simulink model "Senorless"  (R2023a)
settings: Solver=FixedStepDiscrete  StartTime=0.0  StopTime=2  FixedStep=1/FOC_FRQ  RelTol=1e-3
values from neighbouring files (symbols this model uses):
  ADC_REF = 3.6    [Senorless.sldd]
  ADC_SAMPLE_MAX = 32767.0    [Senorless.sldd]
  AMP_GAIN = 32.0    [Senorless.sldd]
  CURR_INPUT = 3276.0    [Senorless.sldd]
  CURR_KI = 380.0    [Senorless.sldd]
  CURR_KP = 0.04    [Senorless.sldd]
  CURR_LIMIT = 1.1    [Senorless.sldd]
  CURR_OVER = 34.0    [Senorless.sldd]
  CURR_POINT_GAIN = 7.0    [Senorless.sldd]
  CURR_STEP = 32760.0    [Senorless.sldd]
  CURR_UNDER = 0.03    [Senorless.sldd]
  CURR_WIDTH = 250.0    [Senorless.sldd]
  FOC_FRQ = 36000.0    [Senorless.sldd]
  GAMMA = 32767.0    [Senorless.sldd]
  HFI_ID = 2.125    [Senorless.sldd]
  IMAX = 34.0    [Senorless.sldd]
  LPF_FRQ = 300.0    [Senorless.sldd]
  MOTOR_DAMPER = 8.3E-7    [Senorless.sldd]
  MOTOR_FLUX = 0.0012713112    [Senorless.sldd]
  MOTOR_INERTIA = 1.02E-6    [Senorless.sldd]
  MOTOR_LS = 1.8E-5    [Senorless.sldd]
  MOTOR_PN = 7.0    [Senorless.sldd]
  MOTOR_RS = 0.065    [Senorless.sldd]
  NS_COMP_UD = 0.531    [Senorless.sldd]
  PLL_LIMIT = 0.95    [Senorless.sldd]
  PLL_WIDTH = 500.0    [Senorless.sldd]
  PWM_FRQ = 96000000.0    [Senorless.sldd]
  RS_HUNT = 0.002    [Senorless.sldd]
  SMOK_FRQ = 1200.0    [Senorless.sldd]
  SPD_LIMIT = 0.8    [Senorless.sldd]
  SPD_LPF_LEVEL = 15.0    [Senorless.sldd]
  SPD_MAX = 8100.0    [Senorless.sldd]
  SPD_MIN = -8100.0    [Senorless.sldd]
  SPD_REDUCE = 380.0    [Senorless.sldd]
  SPD_STEP = 3.0    [Senorless.sldd]
  SPD_WIDTH = 10.0    [Senorless.sldd]
  TS_POINT_GAIN = 10.0    [Senorless.sldd]
  UDC = 17.0    [Senorless.sldd]
  UDC_GAIN = 21.0    [Senorless.sldd]
  UDC_POINT_GAIN = 10.0    [Senorless.sldd]
undefined symbols (not defined in the file or in its folder): curr_q_ki, curr_q_kp, DiscIntNeverNeededParam, magnitude, PLL_LPF_LEVEL, Udc
libraries: simulink x20, slpidlib x5, mcbcontrolslib x4, mcbplantlib x1, autolibpmsminterior x1, autolibpmsmexterior x1, spspowerguiLib x1
(part 2 of 7)

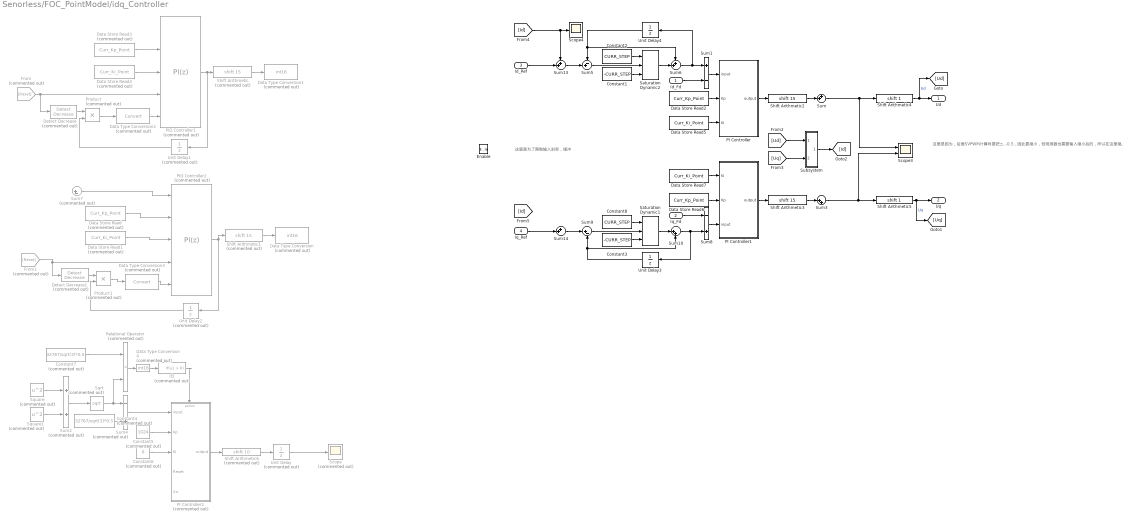
== system Senorless/FOC_PointModel/idq_Controller ==
  note: 这里是为了限制输入斜率，缓冲
  note: 这里是因为，后面SVPWM计算时要把±1映射去±0.5，因此要缩小，但观测器也需要输入缩小后的，所以在这里缩。
  Id_Fd : Inport
  Iq_Fd : Inport  Port=2
  Id_Ref : Inport  Port=3
  Iq_Ref : Inport  Port=4
  Enable : EnablePort  StatesWhenEnabling=reset  PropagateVarSize=During execution
  Constant1 : Constant  Value=-CURR_STEP  OutDataTypeStr=int16
  Constant2 : Constant  Value=CURR_STEP  OutDataTypeStr=int16
  Constant3 : Constant  Value=-CURR_STEP  OutDataTypeStr=int16
  Constant4 : Constant  Commented=on  Value=32767/sqrt(3)*0.5  OutDataTypeStr=int32
  Constant5 : Constant  Commented=on  Value=1024  OutDataTypeStr=int16
  Constant6 : Constant  Commented=on  Value=0  OutDataTypeStr=int16
  Constant7 : Constant  Commented=on  Value=32767/sqrt(3)*0.5  OutDataTypeStr=int32
  Constant8 : Constant  Value=CURR_STEP  OutDataTypeStr=int16
  Data Store Read : DataStoreRead  Commented=on  DataStoreName=Curr_Kp_Point  IndexOptions=Index vector (dialog)  Indices=1  OutputSizes=1
  Data Store Read1 : DataStoreRead  Commented=on  DataStoreName=Curr_Ki_Point  IndexOptions=Index vector (dialog)  Indices=1  OutputSizes=1
  Data Store Read2 : DataStoreRead  DataStoreName=Curr_Kp_Point  IndexOptions=Index vector (dialog)  Indices=1  OutputSizes=1
  Data Store Read3 : DataStoreRead  Commented=on  DataStoreName=Curr_Kp_Point  IndexOptions=Index vector (dialog)  Indices=1  OutputSizes=1
  Data Store Read4 : DataStoreRead  Commented=on  DataStoreName=Curr_Ki_Point  IndexOptions=Index vector (dialog)  Indices=1  OutputSizes=1
  Data Store Read5 : DataStoreRead  DataStoreName=Curr_Ki_Point  IndexOptions=Index vector (dialog)  Indices=1  OutputSizes=1
  Data Store Read6 : DataStoreRead  DataStoreName=Curr_Kp_Point  IndexOptions=Index vector (dialog)  Indices=1  OutputSizes=1
  Data Store Read7 : DataStoreRead  DataStoreName=Curr_Ki_Point  IndexOptions=Index vector (dialog)  Indices=1  OutputSizes=1
  Data Type Conversion : DataTypeConversion  Commented=on  OutDataTypeStr=int16  SaturateOnIntegerOverflow=off  RndMeth=Floor
  Data Type Conversion1 : DataTypeConversion  Commented=on  OutDataTypeStr=int16  SaturateOnIntegerOverflow=off  RndMeth=Floor
  Data Type Conversion2 : DataTypeConversion  Commented=on  SaturateOnIntegerOverflow=off  RndMeth=Floor
  Data Type Conversion3 : DataTypeConversion  Commented=on  SaturateOnIntegerOverflow=off  RndMeth=Floor
  Data Type Conversion4 : DataTypeConversion  Commented=on  OutDataTypeStr=int16  SaturateOnIntegerOverflow=off
  Detect Decrease : simulink/Logic and Bit Operations/Detect Decrease  Commented=on  vinit=0.0  OutDataTypeStr=uint8
  Detect Decrease1 : simulink/Logic and Bit Operations/Detect Decrease  Commented=on  vinit=0.0  OutDataTypeStr=uint8
  From : From  Commented=on  GotoTag=Reset
  From1 : From  Commented=on  GotoTag=Reset
  If2 : If  Commented=on  ShowElse=off
  PI Controller : Subsystem
      settings: MinAlgLoopOccurrences=on
  PI Controller1 : Subsystem
      settings: MinAlgLoopOccurrences=on
  PI Controller2 : Subsystem  Commented=on  TreatAsAtomicUnit=on
      settings: MinAlgLoopOccurrences=on
  PID Controller1 : slpidlib/PID Controller  Commented=on  Controller=PI  Form=Parallel  TimeDomain=Discrete-time  UseExternalTs=off  SampleTime=-1  IntegratorMethod=Forward Euler  FilterMethod=Forward Euler  ControllerParametersSource=external  P=curr_q_kp  I=curr_q_ki  UseKiTs=off  D=0  N=100  UseFilter=on  TunerSelectOption=Transfer Function Based (PID Tuner App)  ZeroCross=off  InitialConditionSource=external  InitialConditionForIntegrator=0  InitialConditionForFilter=0  DifferentiatorICPrevScaledInput=0  ExternalReset=either  TrackingMode=off  Kt=1  LimitOutput=on  SatLimitsSource=internal  UpperSaturationLimit=32767*32767  LowerSaturationLimit=-32767*32767  LinearizeAsGain=on  AntiWindupMode=clamping  Kb=1  LimitIntegrator=on  UpperIntegratorSaturationLimit=32767*32767  LowerIntegratorSaturationLimit=-32767*32767  RndMeth=Zero  SaturateOnIntegerOverflow=on  PGainOutDataTypeStr=int32  PProdOutDataTypeStr=int32  POutMin=[]  POutMax=[]  IGainOutDataTypeStr=int32  IProdOutDataTypeStr=int32  IOutMin=[]  IOutMax=[]  DOutMin=[]  DOutMax=[]  NOutMin=[]  NOutMax=[]  SumOutDataTypeStr=int32  SumOutMin=[]  SumOutMax=[]  SaturationOutDataTypeStr=int32  SaturationOutMin=[]  SaturationOutMax=[]  PParamMin=[]  PParamMax=[]  IParamMin=[]  IParamMax=[]  DParamMin=[]  DParamMax=[]  NParamMin=[]  NParamMax=[]  KbParamMin=[]  KbParamMax=[]  KtParamMin=[]  KtParamMax=[]  KbOutMin=[]  KbOutMax=[]  KtOutMin=[]  KtOutMax=[]  IntegratorOutDataTypeStr=int32  IntegratorOutMin=[]  IntegratorOutMax=[]  FilterOutMin=[]  FilterOutMax=[]  SumI1OutMin=[]  SumI1OutMax=[]  SumI2OutMin=[]  SumI2OutMax=[]  SumI3OutMin=[]  SumI3OutMax=[]  SumI4OutMin=[]  SumI4OutMax=[]  SumDOutMin=[]  SumDOutMax=[]  SumAccumDataTypeStr=int32  DifferentiatorOutMin=[]  DifferentiatorOutMax=[]  FilterDiffOutCoefMin=[]  FilterDiffOutCoefMax=[]  ReciprocalOutMin=[]  ReciprocalOutMax=[]  SumDenOutMin=[]  SumDenOutMax=[]  SumNumOutMin=[]  SumNumOutMax=[]  DivideOutMin=[]  DivideOutMax=[]  UdiffTsProdOutMin=[]  UdiffTsProdOutMax=[]  NTsProdOutMin=[]  NTsProdOutMax=[]  UintegralTsProdOutMin=[]  UintegralTsProdOutMax=[]  UngainTsProdOutMin=[]  UngainTsProdOutMax=[]  ClampingZeroOutDataTypeStr=int32  ClampingZeroOutMin=[]  ClampingZeroOutMax=[]  FilterDenConstantOutDataTypeStr=Inherit: Inherit via back propagation  FilterDenConstantOutMin=[]  FilterDenConstantOutMax=[]  PCopyOutDataTypeStr=Inherit: Inherit via back propagation  PCopyOutMin=[]  PCopyOutMax=[]  NCopyOutDataTypeStr=Inherit: Inherit via back propagation  NCopyOutMin=[]  NCopyOutMax=[]  IntegratorContinuousStateAttributes=''  IntegratorStateMustResolveToSignalObject=off  IntegratorRTWStateStorageClass=Auto  FilterContinuousStateAttributes=''  FilterStateMustResolveToSignalObject=off  FilterRTWStateStorageClass=Auto  ParallelPVariant=ExternalParameters  IdealPVariant=Disabled  IVariant=ExternalParameters  DVariant=Disabled  IntegratorVariant=Discrete  SatVariant=Enabled  AWVariant=DiscClampingParallel  PCopyVariant=Disabled  TRVariant=Disabled  FdbkBlocksVariant=Forward  IdealPFdbkVariant=Disabled  SatFdbkVariant=Disabled  DerivativeFilterVariant=Disabled  NVariant=Disabled  NCopyVariant=Disabled_SignalSpec  FilterICVariant=Disabled  IntegratorICVariant=ExternalICs  ExternalResetVariant=ExternalReset  TRSumVariant=Passthrough  SumFdbkVariant=Disabled  SumVariant=Sum_PI  TsampFilterVariant=InternalTs  TsampNgainVariant=Passthrough  TsampIntegralVariant=Disabled_SignalSpec  ExternalSaturationOutDataTypeStr=int32
  PID Controller2 : slpidlib/PID Controller  Commented=on  Controller=PI  Form=Parallel  TimeDomain=Discrete-time  UseExternalTs=off  SampleTime=-1  IntegratorMethod=Forward Euler  FilterMethod=Forward Euler  ControllerParametersSource=external  P=curr_q_kp  I=curr_q_ki  UseKiTs=off  D=0  N=100  UseFilter=on  TunerSelectOption=Transfer Function Based (PID Tuner App)  ZeroCross=off  InitialConditionSource=external  InitialConditionForIntegrator=0  InitialConditionForFilter=0  DifferentiatorICPrevScaledInput=0  ExternalReset=either  TrackingMode=off  Kt=1  LimitOutput=on  SatLimitsSource=internal  UpperSaturationLimit=32767*32767  LowerSaturationLimit=-32767*32767  LinearizeAsGain=on  AntiWindupMode=none  Kb=1  LimitIntegrator=on  UpperIntegratorSaturationLimit=32767*32767  LowerIntegratorSaturationLimit=-32767*32767  RndMeth=Zero  SaturateOnIntegerOverflow=on  PGainOutDataTypeStr=int32  PProdOutDataTypeStr=int32  POutMin=[]  POutMax=[]  IGainOutDataTypeStr=int32  IProdOutDataTypeStr=int32  IOutMin=[]  IOutMax=[]  DOutMin=[]  DOutMax=[]  NOutMin=[]  NOutMax=[]  SumOutDataTypeStr=int32  SumOutMin=[]  SumOutMax=[]  SaturationOutDataTypeStr=int32  SaturationOutMin=[]  SaturationOutMax=[]  PParamMin=[]  PParamMax=[]  IParamMin=[]  IParamMax=[]  DParamMin=[]  DParamMax=[]  NParamMin=[]  NParamMax=[]  KbParamMin=[]  KbParamMax=[]  KtParamMin=[]  KtParamMax=[]  KbOutMin=[]  KbOutMax=[]  KtOutMin=[]  KtOutMax=[]  IntegratorOutDataTypeStr=int32  IntegratorOutMin=[]  IntegratorOutMax=[]  FilterOutMin=[]  FilterOutMax=[]  SumI1OutMin=[]  SumI1OutMax=[]  SumI2OutMin=[]  SumI2OutMax=[]  SumI3OutMin=[]  SumI3OutMax=[]  SumI4OutMin=[]  SumI4OutMax=[]  SumDOutMin=[]  SumDOutMax=[]  SumAccumDataTypeStr=int32  DifferentiatorOutMin=[]  DifferentiatorOutMax=[]  FilterDiffOutCoefMin=[]  FilterDiffOutCoefMax=[]  ReciprocalOutMin=[]  ReciprocalOutMax=[]  SumDenOutMin=[]  SumDenOutMax=[]  SumNumOutMin=[]  SumNumOutMax=[]  DivideOutMin=[]  DivideOutMax=[]  UdiffTsProdOutMin=[]  UdiffTsProdOutMax=[]  NTsProdOutMin=[]  NTsProdOutMax=[]  UintegralTsProdOutMin=[]  UintegralTsProdOutMax=[]  UngainTsProdOutMin=[]  UngainTsProdOutMax=[]  ClampingZeroOutDataTypeStr=int32  ClampingZeroOutMin=[]  ClampingZeroOutMax=[]  FilterDenConstantOutDataTypeStr=Inherit: Inherit via back propagation  FilterDenConstantOutMin=[]  FilterDenConstantOutMax=[]  PCopyOutDataTypeStr=Inherit: Inherit via back propagation  PCopyOutMin=[]  PCopyOutMax=[]  NCopyOutDataTypeStr=Inherit: Inherit via back propagation  NCopyOutMin=[]  NCopyOutMax=[]  IntegratorContinuousStateAttributes=''  IntegratorStateMustResolveToSignalObject=off  IntegratorRTWStateStorageClass=Auto  FilterContinuousStateAttributes=''  FilterStateMustResolveToSignalObject=off  FilterRTWStateStorageClass=Auto  ParallelPVariant=ExternalParameters  IdealPVariant=Disabled  IVariant=ExternalParameters  DVariant=Disabled  IntegratorVariant=Discrete  SatVariant=Enabled  AWVariant=Passthrough  PCopyVariant=Disabled  TRVariant=Disabled  FdbkBlocksVariant=Forward  IdealPFdbkVariant=Disabled  SatFdbkVariant=Disabled  DerivativeFilterVariant=Disabled  NVariant=Disabled  NCopyVariant=Disabled_SignalSpec  FilterICVariant=Disabled  IntegratorICVariant=ExternalICs  ExternalResetVariant=ExternalReset  TRSumVariant=Passthrough  SumFdbkVariant=Disabled  SumVariant=Sum_PI  TsampFilterVariant=InternalTs  TsampNgainVariant=Passthrough  TsampIntegralVariant=Disabled_SignalSpec  ExternalSaturationOutDataTypeStr=int32
  Product : Product  Commented=on  OutDataTypeStr=int32  RndMeth=Zero
  Product1 : Product  Commented=on  OutDataTypeStr=int32  RndMeth=Zero
  Relational Operator : RelationalOperator  Commented=on  Operator=<  OutDataTypeStr=boolean  RndMeth=Zero  InputSameDT=off
  Saturation Dynamic1 : simulink/Discontinuities/Saturation Dynamic  OutMin=[]  OutMax=[]  OutDataTypeStr=Inherit: Same as second input  OutDataType=fixdt(1, 16)  OutScaling=2^-10  RndMeth=Zero  DoSatur=off
  Saturation Dynamic2 : simulink/Discontinuities/Saturation Dynamic  OutMin=[]  OutMax=[]  OutDataTypeStr=Inherit: Same as second input  OutDataType=fixdt(1, 16)  OutScaling=2^-10  RndMeth=Zero  DoSatur=off
  Scope : Scope  Commented=on
  Scope3 : Scope  NumInputPorts=2
  Scope4 : Scope
  Shift Arithmetic : ArithShift  Commented=on  BitShiftNumber=15
  Shift Arithmetic1 : ArithShift  Commented=on  BitShiftNumber=15
  Shift Arithmetic2 : ArithShift  BitShiftNumber=15
  Shift Arithmetic3 : ArithShift  BitShiftNumber=15
  Shift Arithmetic4 : ArithShift  BitShiftNumber=1
  Shift Arithmetic5 : ArithShift  BitShiftNumber=1
  Shift Arithmetic6 : ArithShift  Commented=on  BitShiftNumber=10
  Sqrt : Sqrt  Commented=on  OutputSignalType=real  RndMeth=Zero
  Square : Math  Commented=on  Operator=square
  Square1 : Math  Commented=on  Operator=square
  Subsystem : Subsystem
  Sum : Sum  Inputs=++|
  Sum1 : Sum  Inputs=+-  AccumDataTypeStr=int32  OutDataTypeStr=int32  RndMeth=Zero
  Sum10 : Sum  Inputs=|++  OutDataTypeStr=int16  RndMeth=Zero
  Sum13 : Sum  Inputs=++|  OutDataTypeStr=int16  RndMeth=Zero
  Sum14 : Sum  Inputs=++|  OutDataTypeStr=int16  RndMeth=Zero
  Sum2 : Sum  Commented=on  RndMeth=Zero
  Sum3 : Sum  Inputs=|++
  Sum4 : Sum  Commented=on  Inputs=-+  RndMeth=Zero
  Sum5 : Sum  Inputs=-+|  AccumDataTypeStr=int16  OutDataTypeStr=int16  RndMeth=Zero
  Sum6 : Sum  Inputs=++|  OutDataTypeStr=int16  RndMeth=Zero
  Sum7 : Sum  Commented=on  Inputs=|+-  AccumDataTypeStr=int32  OutDataTypeStr=int32  RndMeth=Zero
  Sum8 : Sum  Inputs=-+  AccumDataTypeStr=int32  OutDataTypeStr=int32  RndMeth=Zero
  Sum9 : Sum  Inputs=|+-  AccumDataTypeStr=int16  OutDataTypeStr=int16  RndMeth=Zero
  Unit Delay : UnitDelay  Commented=on  SampleTime=-1  HasFrameUpgradeWarning=on
  Unit Delay1 : UnitDelay  Commented=on  SampleTime=-1  HasFrameUpgradeWarning=on
  Unit Delay2 : UnitDelay  Commented=on  SampleTime=-1  HasFrameUpgradeWarning=on
  Unit Delay3 : UnitDelay  SampleTime=-1  HasFrameUpgradeWarning=on
  Unit Delay4 : UnitDelay  SampleTime=-1  HasFrameUpgradeWarning=on
  Ud : Outport  OutputWhenDisabled=reset  InitialOutput=int32(0)
  Uq : Outport  Port=2  OutputWhenDisabled=reset  InitialOutput=int32(0)
  wires:
  Sum7/1 -> PID Controller2/1
  Shift Arithmetic/1 -> Data Type Conversion1/1
  Shift Arithmetic1/1 -> Data Type Conversion/1
  Data Store Read/1 -> PID Controller2/2
  Data Store Read1/1 -> PID Controller2/3
  Data Store Read3/1 -> PID Controller1/2
  Data Store Read4/1 -> PID Controller1/3
  PID Controller1/1 -> Unit Delay1/1, Shift Arithmetic/1
  Unit Delay1/1 -> Product/2
  Detect Decrease/1 -> Product/1
  Product/1 -> Data Type Conversion2/1
  From/1 -> PID Controller1/4, Detect Decrease/1
  Unit Delay2/1 -> Product1/2
  Product1/1 -> Data Type Conversion3/1
  From1/1 -> PID Controller2/4, Detect Decrease1/1
  PID Controller2/1 -> Shift Arithmetic1/1, Unit Delay2/1
  Detect Decrease1/1 -> Product1/1
  Data Type Conversion3/1 -> PID Controller2/5
  PI Controller/1(output) -> Shift Arithmetic2/1
  Data Store Read5/1 -> PI Controller/3(Ki)
  Data Type Conversion2/1 -> PID Controller1/5
  Sum1/1 -> PI Controller/1(input)
  PI Controller1/1(output) -> Shift Arithmetic3/1
  Data Store Read2/1 -> PI Controller/2(Kp)
  Saturation Dynamic2/1 -> Sum6/2
  Unit Delay4/1 -> Sum6/1, Sum5/1
  Sum6/1 -> Unit Delay4/1, Sum1/1
  Constant1/1 -> Saturation Dynamic2/3
  Shift Arithmetic3/1 -> Sum3/1
  Shift Arithmetic4/1 -> [Ud], Ud/1  "Ud"
  Shift Arithmetic5/1 -> [Uq], Uq/1  "Uq"
  Square1/1 -> Sum2/2
  Square/1 -> Sum2/1
  Sum2/1 -> Sqrt/1
  Constant4/1 -> Sum4/2
  Sqrt/1 -> Relational Operator/2, Sum4/1
  Sum4/1 -> PI Controller2/1(input)
  Constant5/1 -> PI Controller2/2(Kp)
  Constant6/1 -> PI Controller2/3(Ki)
  Id_Ref/1 -> Sum13/2
  PI Controller2/1(output) -> Shift Arithmetic6/1
  Unit Delay/1 -> Scope/1
  Constant7/1 -> Relational Operator/1
  Relational Operator/1 -> Data Type Conversion4/1
  Data Type Conversion4/1 -> If2/1
  Shift Arithmetic6/1 -> Unit Delay/1
  Id_Fd/1 -> Sum1/2
  Sum5/1 -> Saturation Dynamic2/2
  Constant2/1 -> Saturation Dynamic2/1
  Sum9/1 -> Saturation Dynamic1/2
  Constant8/1 -> Saturation Dynamic1/1
  Constant3/1 -> Saturation Dynamic1/3
  Data Store Read7/1 -> PI Controller1/1(Ki)
  Data Store Read6/1 -> PI Controller1/2(Kp)
  Sum8/1 -> PI Controller1/3(input)
  Iq_Fd/1 -> Sum8/1
  Saturation Dynamic1/1 -> Sum10/1
  Unit Delay3/1 -> Sum10/2, Sum9/2
  Iq_Ref/1 -> Sum14/2
  Sum10/1 -> Sum8/2, Unit Delay3/1
  Sum13/1 -> Sum5/2
  Sum14/1 -> Sum9/1
  [Ud] -> Subsystem/1(Ud)
  [Uq] -> Subsystem/2(Uq)
  Subsystem/1(-Id) -> [Id]
  [Id] -> Sum13/1, Scope4/1
  If2/1 -> PI Controller2/Action
  Sum/1 -> Shift Arithmetic4/1, Scope3/1
  Sum3/1 -> Shift Arithmetic5/1, Scope3/2
  Shift Arithmetic2/1 -> Sum/2

== system Senorless/FOC_PointModel/sincos_4096 ==
  theta : Inport
  Constant1 : Constant  Value=128  OutDataTypeStr=uint16
  Constant3 : Constant  Value=16384+128  OutDataTypeStr=uint16
  Shift Arithmetic : ArithShift  BitShiftNumber=4
  Shift Arithmetic1 : ArithShift  BitShiftNumber=4
  Sin : Lookup_n-D  NumberOfTableDimensions=1  BreakpointsSpecification=Even spacing  BreakpointsForDimension1=uint16(linspace(0,511,512))  BreakpointsForDimension1DataTypeStr=uint16  IndexSearchMethod=Linear search  BeginIndexSearchUsingPreviousIndexResult=on  UseOneInputPortForAllInputData=on  Table=int16(32767*sin(linspace(0,2*pi,4096)))  TableDataTypeStr=int16  IntermediateResultsDataTypeStr=int32  InterpMethod=Flat  ExtrapMethod=Clip  RemoveProtectionInput=on  ApplyFullPrecisionForLinearInterpolation=on  InternalRulePriority=Speed  OutDataTypeStr=int16  RndMeth=Zero  FractionDataTypeStr=fixdt(1,16,0)  InputSameDT=off
  Sin1 : Lookup_n-D  NumberOfTableDimensions=1  BreakpointsSpecification=Even spacing  BreakpointsForDimension1=uint16(linspace(0,511,512))  BreakpointsForDimension1DataTypeStr=uint16  IndexSearchMethod=Linear search  BeginIndexSearchUsingPreviousIndexResult=on  UseOneInputPortForAllInputData=on  Table=int16(32767*sin(linspace(0,2*pi,4096)))  TableDataTypeStr=int16  IntermediateResultsDataTypeStr=int32  InterpMethod=Flat  ExtrapMethod=Clip  RemoveProtectionInput=on  ApplyFullPrecisionForLinearInterpolation=on  InternalRulePriority=Speed  OutDataTypeStr=int16  RndMeth=Zero  FractionDataTypeStr=fixdt(1,16,0)  InputSameDT=off
  Sin2 : Lookup_n-D  Commented=on  NumberOfTableDimensions=1  BreakpointsSpecification=Even spacing  BreakpointsForDimension1=uint16(linspace(0,511,512))  BreakpointsForDimension1DataTypeStr=uint16  IndexSearchMethod=Linear search  BeginIndexSearchUsingPreviousIndexResult=on  UseOneInputPortForAllInputData=on  Table=|  TableDataTypeStr=int16  IntermediateResultsDataTypeStr=int32  InterpMethod=Flat  ExtrapMethod=Clip  RemoveProtectionInput=on  ApplyFullPrecisionForLinearInterpolation=on  InternalRulePriority=Speed  OutDataTypeStr=int16  RndMeth=Zero  FractionDataTypeStr=fixdt(1,16,0)  InputSameDT=off
      | int16([
      |  0 ,   402 ,   804 ,  1207 ,  1609 , ...
      |       2011 ,  2412 ,  2814 ,  3214 ,  3615 , ...
      |       4015 ,  4414 ,  4812 ,  5210 ,  5607 , ...
      |       6003 ,  6398 ,  6793 ,  7186 ,  7578 , ...
      |       7969 ,  8359 ,  8747 ,  9135 ,  9521 , ...
      |       9905 , 10288 , 10669 , 11049 , 11427 , ...
      |      11804 , 12178 , 12551 , 12922 , 13291 , ...
      |      13658 , 14022 , 14385 , 14746 , 15104 , ...
      |      15460 , 15814 , 16165 , 16514 , 16860 , ...
      |      17204 , 17546 , 17884 , 18220 , 18553 , ...
      |      18884 , 19211 , 19536 , 19857 , 20176 , ...
      |      20492 , 20804 , 21114 , 21420 , 21723 , ...
      |      22023 , 22319 , 22612 , 22902 , 23188 , ...
      |      23470 , 23750 , 24025 , 24297 , 24565 , ...
      |      24830 , 25090 , 25347 , 25601 , 25850 , ...
      |      26095 , 26337 , 26574 , 26808 , 27037 , ...
      |      27263 , 27484 , 27701 , 27914 , 28123 , ...
      |      28327 , 28527 , 28723 , 28915 , 29102 , ...
      |      29285 , 29463 , 29637 , 29806 , 29971 , ...
      |      30132 , 30288 , 30439 , 30586 , 30728 , ...
      |      30865 , 30998 , 31126 , 31250 , 31368 , ...
      |      31482 , 31592 , 31696 , 31796 , 31891 , ...
      |      31981 , 32066 , 32146 , 32222 , 32293 , ...
      |      32359 , 32419 , 32476 , 32527 , 32573 , ...
      |      32614 , 32651 , 32682 , 32709 , 32730 , ...
      |      32747 , 32759 , 32766 , 32767 , 32764 , ...
      |      32756 , 32743 , 32725 , 32703 , 32675 , ...
      |      32642 , 32604 , 32562 , 32514 , 32462 , ...
      |      32405 , 32343 , 32275 , 32204 , 32127 , ...
      |      32045 , 31959 , 31867 , 31771 , 31670 , ...
      |      31565 , 31454 , 31339 , 31219 , 31095 , ...
      |      30965 , 30831 , 30693 , 30549 , 30402 , ...
      |      30249 , 30092 , 29930 , 29764 , 29594 , ...
      |      29419 , 29239 , 29055 , 28867 , 28674 , ...
      |      28478 , 28276 , 28071 , 27861 , 27647 , ...
      |      27429 , 27207 , 26980 , 26750 , 26515 , ...
      |      26277 , 26034 , 25788 , 25538 , 25284 , ...
      |      25026 , 24764 , 24498 , 24229 , 23956 , ...
      |      23680 , 23400 , 23117 , 22830 , 22539 , ...
      |      22245 , 21948 , 21647 , 21344 , 21037 , ...
      |      20726 , 20413 , 20097 , 19777 , 19455 , ...
      |      19130 , 18801 , 18470 , 18136 , 17800 , ...
      |      17461 , 17119 , 16774 , 16427 , 16078 , ...
      |      15726 , 15371 , 15015 , 14656 , 14295 , ...
      |      13931 , 13566 , 13199 , 12829 , 12458 , ...
      |      12085 , 11710 , 11333 , 10954 , 10574 , ...
      |      10192 ,  9809 ,  9424 ,  9038 ,  8650 , ...
      |       8262 ,  7871 ,  7480 ,  7088 ,  6694 , ...
      |       6300 ,  5904 ,  5508 ,  5111 ,  4713 , ...
      |       4314 ,  3915 ,  3515 ,  3114 ,  2713 , ...
      |       2312 ,  1910 ,  1508 ,  1106 ,   704 , ...
      |        301 ,  -100 ,  -503 ,  -905 , -1307 , ...
      |      -1709 , -2111 , -2513 , -2914 , -3315 , ...
      |      -3715 , -4114 , -4513 , -4912 , -5309 , ...
      |      -5706 , -6102 , -6497 , -6891 , -7284 , ...
      |      -7676 , -8067 , -8456 , -8844 , -9231 , ...
      |      -9617 ,-10001 ,-10383 ,-10764 ,-11144 , ...
      |     -11521 ,-11897 ,-12271 ,-12644 ,-13014 , ...
      |     -13383 ,-13749 ,-14113 ,-14475 ,-14835 , ...
      |     -15193 ,-15549 ,-15902 ,-16253 ,-16601 , ...
      |     -16947 ,-17290 ,-17630 ,-17968 ,-18304 , ...
      |     -18636 ,-18966 ,-19293 ,-19616 ,-19937 , ...
      |     -20255 ,-20570 ,-20882 ,-21191 ,-21496 , ...
      |     -21798 ,-22097 ,-22393 ,-22685 ,-22973 , ...
      |     -23259 ,-23541 ,-23819 ,-24093 ,-24364 , ...
      |     -24632 ,-24895 ,-25155 ,-25411 ,-25663 , ...
      |     -25912 ,-26156 ,-26397 ,-26633 ,-26866 , ...
      |     -27094 ,-27318 ,-27538 ,-27755 ,-27966 , ...
      |     -28174 ,-28377 ,-28577 ,-28771 ,-28962 , ...
      |     -29148 ,-29330 ,-29507 ,-29680 ,-29848 , ...
      |     -30012 ,-30171 ,-30326 ,-30476 ,-30622 , ...
      |     -30763 ,-30899 ,-31031 ,-31157 ,-31280 , ...
      |     -31397 ,-31510 ,-31618 ,-31721 ,-31820 , ...
      |     -31914 ,-32003 ,-32087 ,-32166 ,-32240 , ...
      |     -32310 ,-32374 ,-32434 ,-32489 ,-32539 , ...
      |     -32584 ,-32624 ,-32659 ,-32689 ,-32715 , ...
      |     -32735 ,-32750 ,-32761 ,-32767 ,-32767 , ...
      |     -32763 ,-32754 ,-32739 ,-32720 ,-32696 , ...
      |     -32667 ,-32633 ,-32594 ,-32550 ,-32502 , ...
      |     -32448 ,-32390 ,-32326 ,-32258 ,-32185 , ...
      |     -32107 ,-32024 ,-31936 ,-31844 ,-31747 , ...
      |     -31644 ,-31538 ,-31426 ,-31310 ,-31189 , ...
      |     -31063 ,-30932 ,-30797 ,-30657 ,-30513 , ...
      |     -30364 ,-30210 ,-30052 ,-29889 ,-29722 , ...
      |     -29550 ,-29374 ,-29194 ,-29009 ,-28819 , ...
      |     -28626 ,-28428 ,-28225 ,-28019 ,-27808 , ...
      |     -27593 ,-27374 ,-27150 ,-26923 ,-26692 , ...
      |     -26456 ,-26217 ,-25973 ,-25726 ,-25475 , ...
      |     -25219 ,-24961 ,-24698 ,-24432 ,-24161 , ...
      |     -23888 ,-23610 ,-23330 ,-23045 ,-22757 , ...
      |     -22466 ,-22171 ,-21873 ,-21572 ,-21267 , ...
      |     -20959 ,-20648 ,-20334 ,-20017 ,-19697 , ...
      |     -19374 ,-19048 ,-18719 ,-18387 ,-18052 , ...
      |     -17715 ,-17375 ,-17033 ,-16688 ,-16340 , ...
      |     -15990 ,-15637 ,-15282 ,-14925 ,-14566 , ...
      |     -14204 ,-13840 ,-13474 ,-13106 ,-12737 , ...
      |     -12365 ,-11991 ,-11616 ,-11238 ,-10859 , ...
      |     -10479 ,-10097 , -9713 , -9328 , -8941 , ...
      |      -8553 , -8164 , -7774 , -7382 , -6989 , ...
      |      -6596 , -6201 , -5805 , -5409 , -5011 , ...
      |      -4613 , -4214 , -3815 , -3415 , -3014 , ...
      |      -2613 , -2212 , -1810 , -1408 , -1006 , ...
      |       -603 ,  -201 ...
      |     ])
  Sin3 : Lookup_n-D  Commented=on  NumberOfTableDimensions=1  BreakpointsSpecification=Even spacing  BreakpointsForDimension1=uint16(linspace(0,511,512))  BreakpointsForDimension1DataTypeStr=uint16  IndexSearchMethod=Linear search  BeginIndexSearchUsingPreviousIndexResult=on  UseOneInputPortForAllInputData=on  Table=int16(32767*sin(linspace(0,2*pi,512)))  TableDataTypeStr=int16  IntermediateResultsDataTypeStr=int32  InterpMethod=Flat  ExtrapMethod=Clip  RemoveProtectionInput=on  ApplyFullPrecisionForLinearInterpolation=on  InternalRulePriority=Speed  OutDataTypeStr=int16  RndMeth=Zero  FractionDataTypeStr=fixdt(1,16,0)  InputSameDT=off
  Sum1 : Sum  Inputs=|++
  Sum2 : Sum  Inputs=|++
  theta1 : InportShadow
  sin : Outport
  cos : Outport  Port=2
  wires:
  Shift Arithmetic/1 -> Sin1/1
  Sum2/1 -> Shift Arithmetic/1
  Constant3/1 -> Sum2/2
  Shift Arithmetic1/1 -> Sin/1
  theta1/1 -> Sum2/1
  theta/1 -> Sum1/1
  Sin/1 -> sin/1
  Sin1/1 -> cos/1
  Sum1/1 -> Shift Arithmetic1/1
  Constant1/1 -> Sum1/2

== system Senorless/FOC_PointModel/停止等待 ==
  Action Port : ActionPort  InitializeStates=reset  ActionPortLabel=case [ 0 ]:
  Constant1 : Constant  Value=0  OutDataTypeStr=int16
  Constant2 : Constant  Value=0  OutDataTypeStr=uint16
  Constant3 : Constant  Value=0  OutDataTypeStr=int16
  Constant4 : Constant  OutDataTypeStr=int32
  Data Store Write : DataStoreWrite  DataStoreName=NS_Flag  IndexOptions=Index vector (dialog)  Indices=1  OutputSizes=1
  Theta : Outport
  Iq : Outport  Port=2
  Id : Outport  Port=3
  wires:
  Constant1/1 -> Iq/1
  Constant2/1 -> Theta/1
  Constant3/1 -> Id/1
  Constant4/1 -> Data Store Write/1

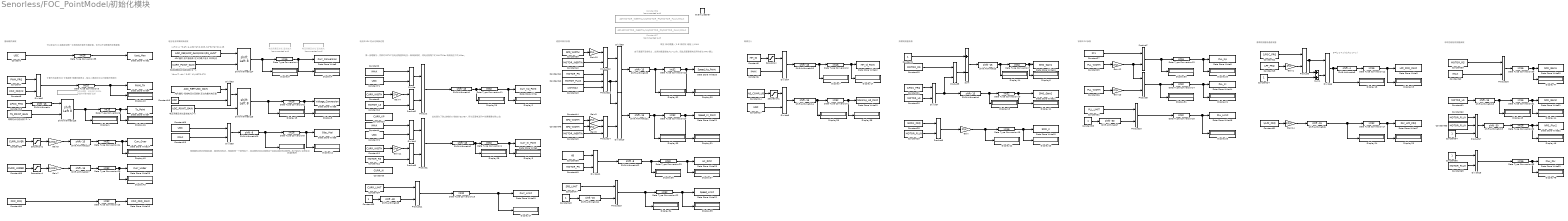
== system Senorless/FOC_PointModel/初始化模块 ==
  note: 非线性磁链观测器参数
  note: 由于速度环没有标幺，出来的是直接放大2^15的，因此后面要把电流环的标幺IMAX算上
  note: 带宽*转动惯量/（1.5*极对数*磁链）/IMAX
  note: 速度环相关系数
  note: 滑模观测器低通滤波器
  note: 锁相环PID参数
  note: 观测器电流电压转换系数，指将电压电流转换到同一个参考系下，如这里电压定点值乘这个后就会换去电流参考：32768/10这种定点
  note: 滑模观测器系数
  note: 高频注入
  note: 电流环KPKI定点化转换过程
  note: 基础硬件参数
  note: 电压电流采集转换系数
  note: 可以在运行init函数前读取一次母线电压值作为确定值，也可以不读取修改字典参数
  note: 此处是为了防止参数为小数放大32767，所以后面电流环PI结果需要左移15位
  note: 第一部理解为，同样的32767在电流角度和电压角度是不一样的概念，这里是做转换用的，将电流视角下的MAX=IMax转到电压下的UMax。
  note: iwf = iw *3.6f / 6.4/32767/0.005 /10*32767=11.25
  note: Vbus = vdc * 3.6f * 41/48=3.075
  note: 计算方式就是PWM计数频率/想要的频率/2，除以二是因为中心计数模式导致的
  note: a=(ω c​ T s​ )/(1+ω c​ T s​ )
  ADC量程*母线电压分压倍数/定义的最大电压值 : Constant  Value=ADC_REF*UDC_GAIN
  ADC量程/放大器倍数/定义的最大电流/采样电流 : Constant  Value=ADC_REF/AMP_GAIN/IMAX/RS_HUNT
  Constant{,17,69,71..72} (5 alike) : Constant  Value=UDC  OutDataTypeStr=single
  Constant{1,24,33,35,48} (5 alike) : Constant  OutDataTypeStr=single
  Constant10 : Constant  Value=MOTOR_LS  OutDataTypeStr=single
  Constant11 : Constant  Value=CURR_WIDTH  OutDataTypeStr=single
  Constant12 : Constant  Value=MOTOR_RS  OutDataTypeStr=single
  Constant{2,4,6,13} (4 alike) : Constant  Value=IMAX  OutDataTypeStr=single
  Constant14 : Constant  Value=NS_COMP_UD  OutDataTypeStr=single
  Constant15 : Constant  Value=MOTOR_RS  OutDataTypeStr=single
  Constant16 : Constant  Value=UDC
  Constant18 : Constant  Value=1/FOC_FRQ  VectorParams1D=off  OutDataTypeStr=double
  Constant19 : Constant  Value=LPF_FRQ
  Constant20 : Constant  Value=MOTOR_LS  OutDataTypeStr=single
  Constant21 : Constant  Value=1/FOC_FRQ  VectorParams1D=off  OutDataTypeStr=double
  Constant22 : Constant  Value=1/FOC_FRQ  VectorParams1D=off  OutDataTypeStr=double
  Constant23 : Constant  Value=CURR_KP  OutDataTypeStr=single
  Constant25 : Constant  Value=PLL_WIDTH
  Constant26 : Constant  Value=PLL_WIDTH
  Constant27 : Constant  Value=2*1  OutDataTypeStr=single
  Constant28 : Constant  Value=SMOK_FRQ
  Constant{29,42,62..63,65} (5 alike) : Constant  Value=MOTOR_FLUX
  Constant3 : Constant  Value=CURR_KI  OutDataTypeStr=single
  Constant30 : Constant  Value=FOC_FRQ  VectorParams1D=off
  Constant31 : Constant  Value=1/LPF_FRQ  VectorParams1D=off  OutDataTypeStr=single
  Constant32 : Constant  Value=PLL_LIMIT
  Constant34 : Constant  Value=CURR_LIMIT  OutDataTypeStr=single
  Constant36 : Constant  Commented=on  Value=40*MOTOR_INERTIA/1.5/MOTOR_PN/MOTOR_FLUX/IMAX  OutDataTypeStr=single
  Constant37 : Constant  Commented=on  Value=40*40*MOTOR_INERTIA/1.5/MOTOR_PN/MOTOR_FLUX/IMAX  OutDataTypeStr=single
  Constant38 : Constant  Value=60  OutDataTypeStr=single
  Constant39 : Constant  Value=SPD_WIDTH
  Constant40 : Constant  Value=MOTOR_INERTIA
  Constant41 : Constant  Value=MOTOR_PN
  Constant43 : Constant  Value=1.5*IMAX
  Constant44 : Constant  Value=SPD_WIDTH
  Constant45 : Constant  Value=MOTOR_INERTIA
  Constant46 : Constant  Value=SPD_WIDTH
  Constant47 : Constant  Value=SPD_LIMIT
  Constant49 : Constant  Value=MOTOR_PN
  Constant5 : Constant  Value=HFI_ID  OutDataTypeStr=single
  Constant50 : Constant  Value=CURR_OVER  VectorParams1D=off
  Constant58 : Constant  Value=CURR_UNDER  VectorParams1D=off
  Constant59 : Constant  Value=MOTOR_RS  OutDataTypeStr=single
  Constant60 : Constant  Value=IMAX
  Constant61 : Constant  Value=MOTOR_LS  OutDataTypeStr=single
  Constant64 : Constant
  Constant66 : Constant
  Constant7 : Constant  Value=PWM_FRQ
  Constant8 : Constant  Value=FOC_FRQ*2  OutDataTypeStr=double
  Constant9 : Constant  Value=CURR_WIDTH  OutDataTypeStr=single
  Data Store Write : DataStoreWrite  DataStoreName=Curr_Kp_Point  IndexOptions=Index vector (dialog)  Indices=1  OutputSizes=1
  Data Store Write1 : DataStoreWrite  DataStoreName=Uout_Max  IndexOptions=Index vector (dialog)  Indices=1  OutputSizes=1
  Data Store Write10 : DataStoreWrite  DataStoreName=SMO_Gain1  IndexOptions=Index vector (dialog)  Indices=1  OutputSizes=1
  Data Store Write11 : DataStoreWrite  DataStoreName=SMO_Gain2  IndexOptions=Index vector (dialog)  Indices=1  OutputSizes=1
  Data Store Write12 : DataStoreWrite  DataStoreName=HFI_Id_Point  IndexOptions=Index vector (dialog)  Indices=1  OutputSizes=1
  Data Store Write13 : DataStoreWrite  DataStoreName=NScomp_Ud_Point  IndexOptions=Index vector (dialog)  Indices=1  OutputSizes=1
  Data Store Write14 : DataStoreWrite  DataStoreName=PLL_Ki  IndexOptions=Index vector (dialog)  Indices=1  OutputSizes=1
  Data Store Write15 : DataStoreWrite  DataStoreName=SMO_K  IndexOptions=Index vector (dialog)  Indices=1  OutputSizes=1
  Data Store Write16 : DataStoreWrite  DataStoreName=FOC_FRQ_Point  IndexOptions=Index vector (dialog)  Indices=1  OutputSizes=1
  Data Store Write17 : DataStoreWrite  DataStoreName=DIV_LPF_FRQ  IndexOptions=Index vector (dialog)  Indices=1  OutputSizes=1
  Data Store Write18 : DataStoreWrite  DataStoreName=PLL_Limit  IndexOptions=Index vector (dialog)  Indices=1  OutputSizes=1
  Data Store Write19 : DataStoreWrite  DataStoreName=Curr_Limit  IndexOptions=Index vector (dialog)  Indices=1  OutputSizes=1
  Data Store Write2 : DataStoreWrite  DataStoreName=Curr_Ki_Point  IndexOptions=Index vector (dialog)  Indices=1  OutputSizes=1
  Data Store Write20 : DataStoreWrite  DataStoreName=Speed_Kp_Point  IndexOptions=Index vector (dialog)  Indices=1  OutputSizes=1
  Data Store Write21 : DataStoreWrite  DataStoreName=Speed_Ki_Point  IndexOptions=Index vector (dialog)  Indices=1  OutputSizes=1
  Data Store Write22 : DataStoreWrite  DataStoreName=Speed_Limit  IndexOptions=Index vector (dialog)  Indices=1  OutputSizes=1
  Data Store Write23 : DataStoreWrite  DataStoreName=Hz_RPM  IndexOptions=Index vector (dialog)  Indices=1  OutputSizes=1
  Data Store Write24 : DataStoreWrite  DataStoreName=Curr_Over  IndexOptions=Index vector (dialog)  Indices=1  OutputSizes=1
  Data Store Write29 : DataStoreWrite  DataStoreName=Curr_Under  IndexOptions=Index vector (dialog)  Indices=1  OutputSizes=1
  Data Store Write3 : DataStoreWrite  DataStoreName=LPF_FRQ_Point  IndexOptions=Index vector (dialog)  Indices=1  OutputSizes=1
  Data Store Write30 : DataStoreWrite  DataStoreName=NFO_Gain1  IndexOptions=Index vector (dialog)  Indices=1  OutputSizes=1
  Data Store Write31 : DataStoreWrite  DataStoreName=NFO_Gain2  IndexOptions=Index vector (dialog)  Indices=1  OutputSizes=1
  Data Store Write32 : DataStoreWrite  DataStoreName=NFO_Flux2  IndexOptions=Index vector (dialog)  Indices=1  OutputSizes=1
  Data Store Write33 : DataStoreWrite  DataStoreName=Flux_Div  IndexOptions=Index vector (dialog)  Indices=1  OutputSizes=1
  Data Store Write4 : DataStoreWrite  DataStoreName=PWM_TH  IndexOptions=Index vector (dialog)  Indices=1  OutputSizes=1
  Data Store Write5 : DataStoreWrite  DataStoreName=Curr_Conversion  IndexOptions=Index vector (dialog)  Indices=1  OutputSizes=1
  Data Store Write6 : DataStoreWrite  DataStoreName=Voltage_Conversion  IndexOptions=Index vector (dialog)  Indices=1  OutputSizes=1
  Data Store Write7 : DataStoreWrite  Priority=-1  DataStoreName=Ts_Point  IndexOptions=Index vector (dialog)  Indices=1  OutputSizes=1
  Data Store Write8 : DataStoreWrite  DataStoreName=PLL_Kp  IndexOptions=Index vector (dialog)  Indices=1  OutputSizes=1
  Data Store Write9 : DataStoreWrite  DataStoreName=Obs_VtoI  IndexOptions=Index vector (dialog)  Indices=1  OutputSizes=1
  Data Type Conversion{1,9..11,14,16..19,22,24,29} (12 alike) : DataTypeConversion  OutDataTypeStr=int32  RndMeth=Nearest  SaturateOnIntegerOverflow=off
  Data Type Conversion{2,12,15,30..33} (7 alike) : DataTypeConversion  OutDataTypeStr=int16  RndMeth=Ceiling  SaturateOnIntegerOverflow=off
  Data Type Conversion{3..6,8,13,35} (7 alike) : DataTypeConversion  OutDataTypeStr=int16  RndMeth=Nearest  SaturateOnIntegerOverflow=off
  Data Type Conversion{7,20..21,23} (4 alike) : DataTypeConversion  OutDataTypeStr=int32  RndMeth=Ceiling  SaturateOnIntegerOverflow=off
  Display{1..40,43..48,50..51} (48 alike) : Display
  Divide{,1..2,4..9,11,15} (11 alike) : Product  Inputs=*/
  Divide10 : Product  Inputs=/*
  Divide3 : Product  Inputs=*/  RndMeth=Zero
  Event Listener : EventListener  DisableCoverage=on  EventName=reset
  Gain{,1,3..4,9..13} (9 alike) : Gain  Gain=2*pi
  Gain14 : Gain  Gain=1/2/pi
  Gain5 : Gain  Gain=1/IMAX
  Gain7 : Gain  Gain=1/IMAX
  Product{,1..3,5..12,15..16} (14 alike) : Product
  Product13 : Product  Inputs=3
  Product14 : Product  Inputs=3
  Product17 : Product  Inputs=3
  Saturation : Saturate  UpperLimit=IMAX  LowerLimit=-IMAX
  Saturation1 : Saturate  UpperLimit=UDC/2  LowerLimit=-UDC/2
  Saturation2 : Saturate  UpperLimit=IMAX  LowerLimit=-IMAX
  Saturation4 : Saturate  UpperLimit=IMAX  LowerLimit=-IMAX
  Shift Arithmetic{,1..4,6,9..11,13..14,17..18,21} (14 alike) : ArithShift  BitShiftNumber=-15
  Shift Arithmetic12 : ArithShift  BitShiftNumber=-8
  Shift Arithmetic19 : ArithShift  BitShiftNumber=-30
  Shift Arithmetic20 : ArithShift  BitShiftNumber=-8
  Shift Arithmetic24 : ArithShift  BitShiftNumberSource=Input port  BitShiftNumber=8  BitShiftDirection=Left
      settings: InputPortMap=u0,p1
  Shift Arithmetic25 : ArithShift  BitShiftNumberSource=Input port  BitShiftNumber=8  BitShiftDirection=Left
      settings: InputPortMap=u0,p1
  Shift Arithmetic26 : ArithShift  BitShiftNumberSource=Input port  BitShiftNumber=8  BitShiftDirection=Left
      settings: InputPortMap=u0,p1
  Shift Arithmetic5 : ArithShift  BitShiftNumber=-4
  Shift Arithmetic7 : ArithShift  BitShiftNumber=-30
  Shift Arithmetic8 : ArithShift  BitShiftNumber=-30
  Sum : Sum  Inputs=+-
  Sum1 : Sum
  周期定点化适当放大2^n : Constant  Value=TS_POINT_GAIN
  电压采集定点化 适当放大 : ArithShift  Commented=on  BitShiftNumber=-UDC_POINT_GAIN  DiagnosticForOORShift=Error
  电压采集定点化适当放大2^n : Constant  Value=UDC_POINT_GAIN
  电流采集定点化 适当放大 : ArithShift  Commented=on  BitShiftNumber=-CURR_POINT_GAIN  DiagnosticForOORShift=Error
  电流采集定点化适当放大2^n : Constant  Value=CURR_POINT_GAIN
  适当调整，此处放大1024 : ArithShift  Commented=on  BitShiftNumber=-TS_POINT_GAIN  DiagnosticForOORShift=Error
  wires:
  Constant2/1 -> Divide/1
  Constant71/1 -> Divide/2
  Divide/1 -> Product/1
  Data Type Conversion11/1 -> Display2/1, Data Store Write/1
  Constant/1 -> Data Type Conversion35/1
  Constant10/1 -> Product2/2
  Data Type Conversion4/1 -> Display4/1, Data Store Write5/1
  ADC量程/放大器倍数/定义的最大电流/采样电流/1 -> Shift Arithmetic24/1
  Shift Arithmetic24/1 -> Display9/1, Data Type Conversion4/1
  Data Type Conversion5/1 -> Display5/1, Data Store Write6/1
  ADC量程*母线电压分压倍数/定义的最大电压值/1 -> Divide3/1
  Constant16/1 -> Divide3/2
  Divide3/1 -> Shift Arithmetic25/1
  Shift Arithmetic1/1 -> Display29/1, Data Type Conversion11/1
  Data Type Conversion8/1 -> Display12/1, Data Store Write9/1
  Data Type Conversion3/1 -> Display10/1, Data Store Write4/1
  Data Type Conversion6/1 -> Display16/1, Data Store Write7/1
  Constant7/1 -> Divide2/1
  Shift Arithmetic/1 -> Shift Arithmetic26/1
  Constant18/1 -> Shift Arithmetic/1
  Divide2/1 -> Data Type Conversion3/1
  Shift Arithmetic26/1 -> Display1/1, Data Type Conversion6/1
  Constant8/1 -> Divide2/2
  Data Type Conversion9/1 -> Display6/1, Data Store Write10/1
  Divide5/1 -> Shift Arithmetic20/1
  Constant69/1 -> Divide5/1
  Constant13/1 -> Divide5/2
  Constant21/1 -> Divide7/1
  Constant20/1 -> Divide7/2
  Divide7/1 -> Product5/2, Shift Arithmetic4/1
  Shift Arithmetic2/1 -> Display28/1, Data Type Conversion1/1
  Constant12/1 -> Product3/2
  Divide1/1 -> Product1/1
  Constant4/1 -> Divide1/1
  Constant72/1 -> Divide1/2
  Data Type Conversion1/1 -> Display3/1, Data Store Write2/1
  Shift Arithmetic25/1 -> Data Type Conversion5/1, Display15/1
  Data Type Conversion10/1 -> Display11/1, Data Store Write11/1
  Shift Arithmetic3/1 -> Display14/1, Data Type Conversion9/1
  Shift Arithmetic4/1 -> Display13/1, Data Type Conversion10/1
  Sum/1 -> Shift Arithmetic3/1
  Constant1/1 -> Sum/1
  Product5/1 -> Sum/2
  Constant15/1 -> Product5/1
  Data Type Conversion12/1 -> Display19/1, Data Store Write3/1
  Shift Arithmetic5/1 -> Data Type Conversion12/1
  Sum1/1 -> Divide6/2
  Constant24/1 -> Sum1/2
  Divide6/1 -> Display18/1, Shift Arithmetic5/1
  Constant27/1 -> Product7/1
  Product7/1 -> Display50/1, Data Type Conversion13/1
  Product8/1 -> Display51/1, Data Type Conversion14/1
  Data Type Conversion13/1 -> Display20/1, Data Store Write8/1
  Data Type Conversion14/1 -> Display21/1, Data Store Write14/1
  Constant28/1 -> Product9/1
  Constant29/1 -> Product9/2
  Gain/1 -> Data Type Conversion15/1, Display22/1
  Data Type Conversion15/1 -> Data Store Write15/1, Display23/1
  Data Type Conversion16/1 -> Data Store Write16/1
  Constant30/1 -> Data Type Conversion16/1
  Product2/1 -> Product/2
  Product3/1 -> Product1/2
  Shift Arithmetic6/1 -> Display24/1, Data Type Conversion17/1
  Constant31/1 -> Gain14/1
  Data Type Conversion17/1 -> Display25/1, Data Store Write17/1
  电流采集定点化适当放大2^n/1 -> Shift Arithmetic24/2
  电压采集定点化适当放大2^n/1 -> Shift Arithmetic25/2
  周期定点化适当放大2^n/1 -> Shift Arithmetic26/2
  Constant32/1 -> Product10/1
  Constant33/1 -> Shift Arithmetic7/1
  Shift Arithmetic7/1 -> Product10/2
  Product10/1 -> Data Type Conversion18/1
  Data Type Conversion18/1 -> Display26/1, Data Store Write18/1
  Shift Arithmetic8/1 -> Product11/2
  Constant34/1 -> Product11/1
  Constant35/1 -> Shift Arithmetic8/1
  Product11/1 -> Data Type Conversion19/1
  Data Type Conversion19/1 -> Display27/1, Data Store Write19/1
  Product9/1 -> Gain/1
  Shift Arithmetic21/1 -> Data Type Conversion20/1, Display33/1
  Shift Arithmetic9/1 -> Data Type Conversion21/1, Display32/1
  Constant39/1 -> Gain10/1
  Constant40/1 -> Product12/2
  Constant42/1 -> Product13/2
  Constant43/1 -> Product13/3
  Product12/1 -> Divide9/1
  Product13/1 -> Divide10/1, Divide9/2
  Constant44/1 -> Gain3/1
  Constant45/1 -> Product14/3
  Constant46/1 -> Gain9/1
  Product14/1 -> Divide10/2
  Data Type Conversion21/1 -> Display30/1, Data Store Write20/1
  Data Type Conversion20/1 -> Display31/1, Data Store Write21/1
  Product15/1 -> Display34/1, Data Type Conversion22/1
  Shift Arithmetic11/1 -> Product15/2
  Constant47/1 -> Product15/1
  Constant48/1 -> Shift Arithmetic11/1
  Data Type Conversion22/1 -> Data Store Write22/1, Display35/1
  Constant41/1 -> Product13/1
  Divide11/1 -> Shift Arithmetic12/1
  Shift Arithmetic12/1 -> Display36/1, Data Type Conversion23/1
  Data Type Conversion23/1 -> Display37/1, Data Store Write23/1
  Constant49/1 -> Divide11/2
  Constant38/1 -> Divide11/1
  Constant50/1 -> Saturation2/1
  Shift Arithmetic13/1 -> Data Type Conversion24/1
  Data Type Conversion24/1 -> Display40/1, Data Store Write24/1
  Product6/1 -> Sum1/1, Divide6/1
  Saturation2/1 -> Gain5/1
  Gain5/1 -> Shift Arithmetic13/1
  Data Type Conversion29/1 -> Display43/1, Data Store Write29/1
  Shift Arithmetic17/1 -> Data Type Conversion29/1
  Gain7/1 -> Shift Arithmetic17/1
  Saturation4/1 -> Gain7/1
  Constant58/1 -> Saturation4/1
  Product16/1 -> Data Type Conversion30/1
  Data Type Conversion30/1 -> Display47/1, Data Store Write30/1
  Constant59/1 -> Product16/1
  Constant60/1 -> Product16/2
  Data Type Conversion31/1 -> Display44/1, Data Store Write31/1
  Shift Arithmetic18/1 -> Data Type Conversion31/1, Display45/1
  Constant61/1 -> Shift Arithmetic18/1
  Constant62/1 -> Product17/1
  Product17/1 -> Shift Arithmetic19/1
  Shift Arithmetic19/1 -> Data Type Conversion32/1
  Data Type Conversion32/1 -> Display46/1, Data Store Write32/1
  Constant63/1 -> Product17/2
  Constant64/1 -> Product17/3
  Constant65/1 -> Divide15/2
  Constant66/1 -> Divide15/1
  Divide15/1 -> Data Type Conversion33/1
  Data Type Conversion33/1 -> Display48/1, Data Store Write33/1
  Shift Arithmetic20/1 -> Display8/1, Data Type Conversion8/1
  Divide10/1 -> Shift Arithmetic21/1
  Product/1 -> Shift Arithmetic1/1
  Product1/1 -> Shift Arithmetic2/1
  Divide9/1 -> Shift Arithmetic9/1
  Constant9/1 -> Gain4/1
  Constant11/1 -> Gain11/1
  Gain3/1 -> Product14/1
  Gain9/1 -> Product14/2
  Gain10/1 -> Product12/1
  Constant22/1 -> Product6/1
  Constant25/1 -> Gain12/1
  Constant26/1 -> Gain13/1
  Constant19/1 -> Gain1/1
  Gain1/1 -> Product6/2
  Gain4/1 -> Product2/1
  Gain11/1 -> Product3/1
  Gain12/1 -> Product8/1, Product7/2
  Gain13/1 -> Product8/2
  Gain14/1 -> Shift Arithmetic6/1
  Data Type Conversion35/1 -> Data Store Write1/1
  Constant5/1 -> Saturation/1
  Saturation/1 -> Divide4/1
  Constant6/1 -> Divide4/2
  Divide4/1 -> Shift Arithmetic10/1
  Data Type Conversion2/1 -> Display17/1, Data Store Write12/1
  Shift Arithmetic10/1 -> Data Type Conversion2/1, Display7/1
  Constant14/1 -> Saturation1/1
  Saturation1/1 -> Divide8/1
  Constant17/1 -> Divide8/2
  Divide8/1 -> Shift Arithmetic14/1
  Shift Arithmetic14/1 -> Display39/1, Data Type Conversion7/1
  Data Type Conversion7/1 -> Display38/1, Data Store Write13/1
